simulink model "velocitycontrolwitherror"  (R2025b)
settings: Solver=VariableStepAuto  StartTime=0.0  StopTime=10.0  RelTol=1e-3
values from neighbouring files (symbols this model uses):
  K = 1.375    [VelocityvsModel.m]
  Kp = 3    [VelocityvsModel.m]
  sigma = 14    [VelocityvsModel.m]
libraries: simulink x1
settings Model: Creator=jschw  LastModifiedBy=jschw

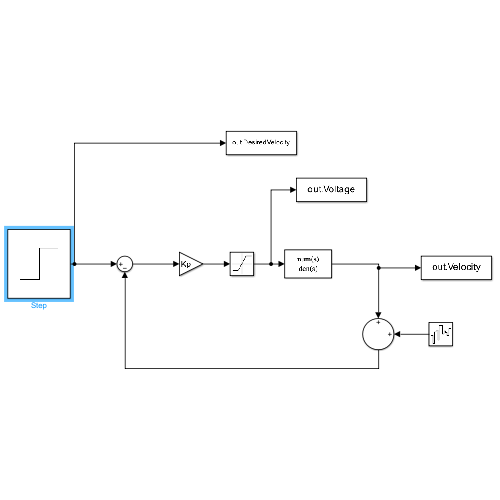
[thumbnail: Simulink's stored preview of the top-level diagram]
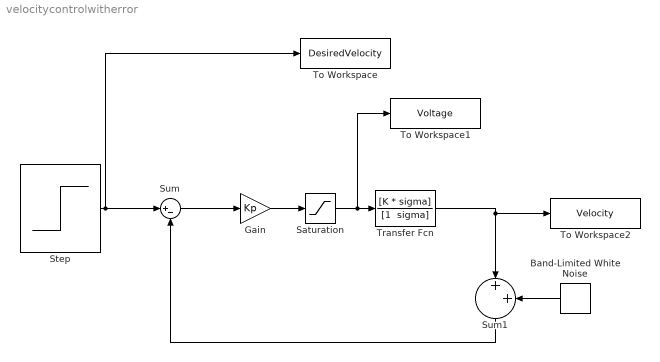
== system velocitycontrolwitherror ==
  Band-Limited White Noise : simulink/Sources/Band-Limited White Noise  Cov=[0.001]  Ts=0.01  seed=[23341]
  Gain : Gain  Gain=Kp
  Saturation : Saturate  UpperLimit=7.5  LowerLimit=-7.5
  Step : Step  Time=2.48  After=2  SampleTime=0
  Sum : Sum  Inputs=|+-
  Sum1 : Sum  Inputs=|++
  To Workspace : ToWorkspace  VariableName=DesiredVelocity  SaveFormat=Timeseries  SampleTime=-1
  To Workspace1 : ToWorkspace  VariableName=Voltage  SaveFormat=Timeseries  SampleTime=-1
  To Workspace2 : ToWorkspace  VariableName=Velocity  SaveFormat=Timeseries  SampleTime=-1
  Transfer Fcn : TransferFcn  Numerator=[K * sigma]  Denominator="[1  sigma]"
  wires:
  Step/1 -> To Workspace/1, Sum/1
  Transfer Fcn/1 -> To Workspace2/1, Sum1/1
  Sum1/1 -> Sum/2
  Band-Limited White Noise/1 -> Sum1/2
  Saturation/1 -> To Workspace1/1, Transfer Fcn/1
  Gain/1 -> Saturation/1
  Sum/1 -> Gain/1
